simulink library "DYN_MAG"  (Simulink 8.8)
settings: Solver=ode45  StartTime=0.0  StopTime=10.0  RelTol=1e-3  EnableMultiTasking=on
undefined symbols (not defined in the file): DYN_SC_par
libraries: LIB_ROT x5, LIB_ENV x1
settings Model: Creator=alger  LastModifiedBy=alger

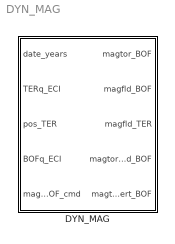
== system DYN_MAG ==
  DYN_MAG : Subsystem

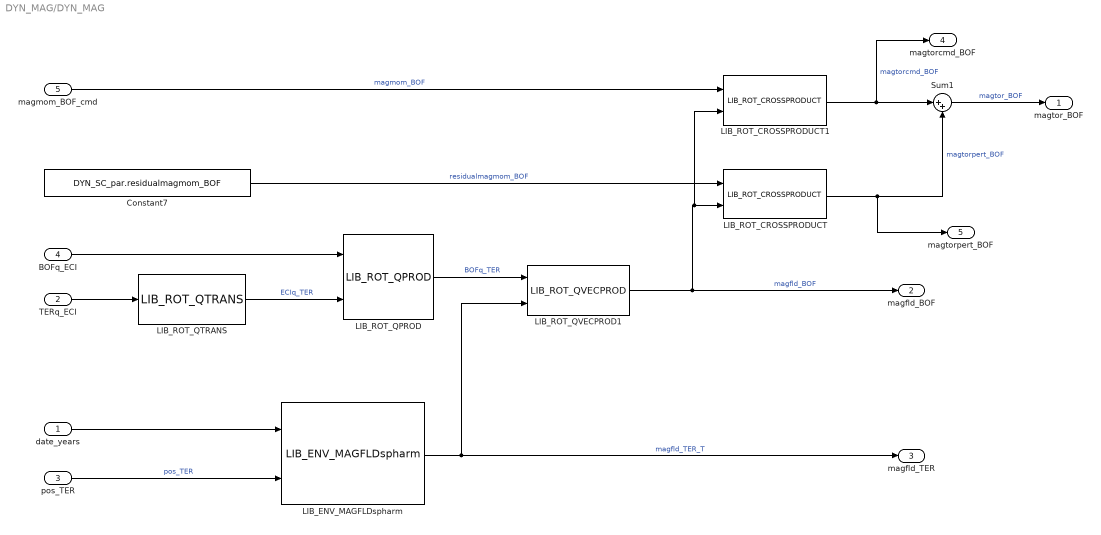
== system DYN_MAG/DYN_MAG ==
  date_years : Inport
  TERq_ECI : Inport  Port=2
  pos_TER : Inport  Port=3
  BOFq_ECI : Inport  Port=4
  magmom_BOF_cmd : Inport  Port=5
  Constant7 : Constant  Value=DYN_SC_par.residualmagmom_BOF
  LIB_ENV_MAGFLDspharm : LIB_ENV/LIB_ENV_MAGFLDspharm  maxDegree=DYN_MAG_par.max_degree  re_cst=CONSTANTS_par.r_earth  Gnm=DYN_MAG_par.Gnm  Hnm=DYN_MAG_par.Hnm  Gnm_dot=DYN_MAG_par.GnmDot  Hnm_dot=DYN_MAG_par.HnmDot  basedate_years=DYN_MAG_par.basedate
  LIB_ROT_CROSSPRODUCT : LIB_ROT/LIB_ROT_CROSSPRODUCT
  LIB_ROT_CROSSPRODUCT1 : LIB_ROT/LIB_ROT_CROSSPRODUCT
  LIB_ROT_QPROD : LIB_ROT/LIB_ROT_QPROD
  LIB_ROT_QTRANS : LIB_ROT/LIB_ROT_QTRANS
  LIB_ROT_QVECPROD1 : LIB_ROT/LIB_ROT_QVECPROD
  Sum1 : Sum  Inputs=|++
  magtor_BOF : Outport
  magfld_BOF : Outport  Port=2
  magfld_TER : Outport  Port=3
  magtorcmd_BOF : Outport  Port=4
  magtorpert_BOF : Outport  Port=5
  wires:
  BOFq_ECI/1 -> LIB_ROT_QPROD/1
  TERq_ECI/1 -> LIB_ROT_QTRANS/1
  pos_TER/1 -> LIB_ENV_MAGFLDspharm/2  "pos_TER"
  date_years/1 -> LIB_ENV_MAGFLDspharm/1
  LIB_ENV_MAGFLDspharm/1 -> LIB_ROT_QVECPROD1/2, magfld_TER/1  "magfld_TER_T"
  Constant7/1 -> LIB_ROT_CROSSPRODUCT/1  "residualmagmom_BOF"
  LIB_ROT_QPROD/1 -> LIB_ROT_QVECPROD1/1  "BOFq_TER"
  LIB_ROT_CROSSPRODUCT/1 -> magtorpert_BOF/1, Sum1/2  "magtorpert_BOF"
  LIB_ROT_QTRANS/1 -> LIB_ROT_QPROD/2  "ECIq_TER"
  LIB_ROT_QVECPROD1/1 -> magfld_BOF/1, LIB_ROT_CROSSPRODUCT1/2, LIB_ROT_CROSSPRODUCT/2  "magfld_BOF"
  Sum1/1 -> magtor_BOF/1  "magtor_BOF"
  magmom_BOF_cmd/1 -> LIB_ROT_CROSSPRODUCT1/1  "magmom_BOF"
  LIB_ROT_CROSSPRODUCT1/1 -> magtorcmd_BOF/1, Sum1/1  "magtorcmd_BOF"
